simulink model "RoomTemperature"  (R2024a)
settings: Solver=VariableStepAuto  StartTime=0.0  StopTime=T  MaxStep=MaxStep  RelTol=RelTol
values from neighbouring files (symbols this model uses):
  J = 20    [Init.m]
  parameters = [a;Tr;Tdelta;Tmin;Tmax]    [Init.m]
  T = 10    [Init.m]
  xInitial = 55    [Init.m]
  xInitialFsm = 0    [Init.m]
libraries: HyEQ_Library x2, SignalEditorBlockLib x1
settings Model: Creator=venkat  LastModifiedBy=venkat

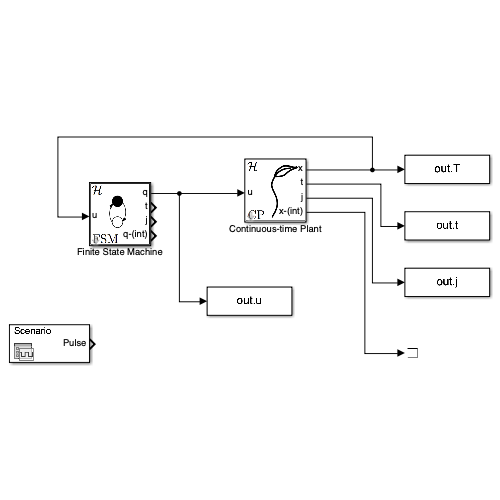
[thumbnail: Simulink's stored preview of the top-level diagram]
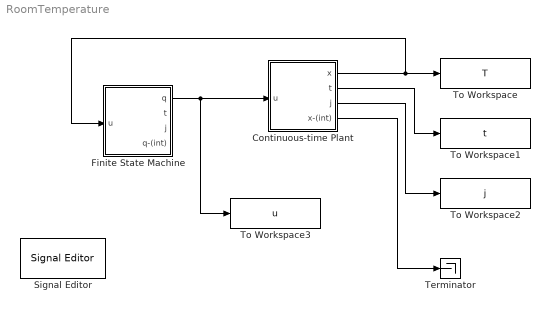
== system RoomTemperature ==
  Continuous-time Plant : Subsystem  LoadFcn=set_param(gcb,'LinkStatus','none')  mask(Continuous Process){z0=xInitial, input_dim=1, parameters=parameters, T=T}
      mask prompts: z0 "Initial State (column vector)"; input_dim "Input dimension (nonnegative integer)"; T "Flow Horizon (nonnegative real)"
      mask help:
      | To define the continuous process:
      | 1. Select the block,
      | 2. "Look inside" the block: Either open the context menu and select Mask > Look Under Mask, or click the arrow in the bottom-left corner of the block.
      | 3. Edit the "flow map f" block to define the continuous dynamics.
      | 4. Edit the "flow set C" block to define the region where the continuous process is allowed to flow.
      mask init:
      | state_dim = size(z0, 1);
      settings: CopyFcn=|
      | set_param(gcb,'LinkStatus','none'),
      | set_param(gcs, 'MaxStep', 'MaxStep', 'RelTol', 'RelTol','StopTime', 'T')
      mask Help: eval hybrid.internal.openHelp('Example_vehicle_on_path')
      mask TypeOptions T: Integrator System/T
      mask DialogControl Control2 Prompt: CPS Components Documentation
      mask DialogControl Control2 Callback: hybrid.internal.openHelp('CPS_Components')
      mask DialogControl ParameterGroupVar Prompt: Configuration
      mask Display:
      | image('Cplant.jpg')
      | port_label('output', 1, 'x')
      | port_label('output', 2, 't')
      | port_label('output', 3, 'j')
      | port_label('output', 4, 'x-(int)')
      | port_label('input', 1, 'u')
  Finite State Machine : Subsystem  LoadFcn=set_param(gcb,'LinkStatus','none')  mask(Finite State Machine (FSM)){q0=xInitialFsm, input_dim=1, T=T, J=J}
      mask prompts: q0 "Initial state (column vector)"; input_dim "Input dimension (nonnegative integer)"; T "Flow Horizon (nonnegative real)"; J "Jump Horizon (nonnegative integer)"
      mask help:
      | To define the FSM:
      | 1. Select the block,
      | 2. "Look inside" the block: Either open the context menu and select Mask > Look Under Mask, or click the arrow in the bottom-left corner of the block.
      | 3. Edit the flow set C, jump set D, and jump map g.
      mask init:
      | state_dim = numel(q0);
      settings: CopyFcn=|
      | set_param(gcb,'LinkStatus','none'),
      | set_param(gcs, 'MaxStep', 'MaxStep', 'RelTol', 'RelTol','StopTime', 'T')
      mask Help: eval hybrid.internal.openHelp('CPS_finite_state_machine')
      mask TypeOptions T: Integrator System/T
      mask TypeOptions J: Integrator System/J
      mask DialogControl Control2 Prompt: CPS Components Documentation
      mask DialogControl Control2 Callback: hybrid.internal.openHelp('CPS_Components')
      mask DialogControl Container4 Prompt: Configuration
      mask Display:
      | image('FSM.jpg')
      | port_label('output', 1, 'q')
      | port_label('output', 2, 't')
      | port_label('output', 3, 'j')
      | port_label('output', 4, 'q-(int)')
      | port_label('input', 1, 'u')
  Signal Editor : SignalEditorBlockLib/Signal Editor  FileName=pulse_signal.mat  ActiveScenario=Scenario  ActiveSignal=Pulse  IsBus=off  OutputBusObjectStr=Bus: BusObject  SampleTime=0  Interpolate=off  ZeroCross=off  OutputAfterFinalValue=Setting to zero  Unit=inherit  PreserveSignalName=on  ApplySigPropsToAllScenarios=on  ApplySigPropsToAllSignals=off
  Terminator : Terminator
  To Workspace : ToWorkspace  VariableName=T  SampleTime=-1
  To Workspace1 : ToWorkspace  VariableName=t  SampleTime=-1
  To Workspace2 : ToWorkspace  VariableName=j  SampleTime=-1
  To Workspace3 : ToWorkspace  VariableName=u  SampleTime=-1
  wires:
  Continuous-time Plant/1(x) -> Finite State Machine/1(u), To Workspace/1
  Continuous-time Plant/2(t) -> To Workspace1/1
  Continuous-time Plant/3(j) -> To Workspace2/1
  Continuous-time Plant/4(x-(int)) -> Terminator/1
  Finite State Machine/1(q) -> To Workspace3/1, Continuous-time Plant/1(u)

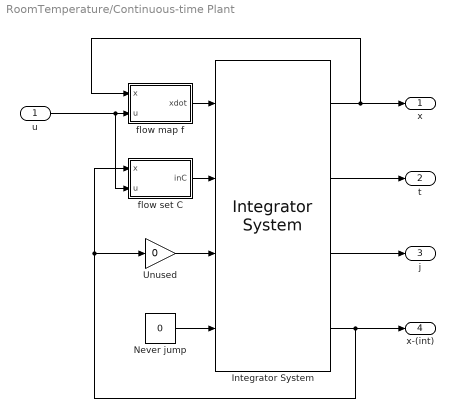
== system RoomTemperature/Continuous-time Plant ==
  u : Inport  PortDimensions=input_dim
  Integrator System : HyEQ_Library/Other/Integrator System  Priority=2  T=T  J=1  x0=z0  rule=1
      settings: SourceProductName=Hybrid Equations Toolbox
  Never jump : Constant  Value=0
  Unused : Gain  Gain=0
  flow map f : MATLAB Function  TreatAsAtomicUnit=on
  flow set C : MATLAB Function  TreatAsAtomicUnit=on
  x : Outport  PortDimensions=state_dim
  t : Outport  Port=2  PortDimensions=1
  j : Outport  Port=3  PortDimensions=1
  x-(int) : Outport  Port=4  PortDimensions=state_dim
  wires:
  Unused/1 -> Integrator System/3
  Never jump/1 -> Integrator System/4
  u/1 -> flow map f/2(u), flow set C/2(u)
  Integrator System/3 -> j/1
  Integrator System/2 -> t/1
  flow set C/1(inC) -> Integrator System/2
  Integrator System/1 -> x/1, flow map f/1(x)
  Integrator System/4 -> x-(int)/1, flow set C/1(x), Unused/1
  flow map f/1(xdot) -> Integrator System/1

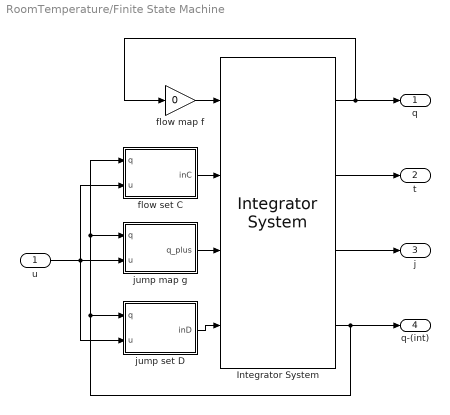
== system RoomTemperature/Finite State Machine ==
  u : Inport  PortDimensions=input_dim
  Integrator System : HyEQ_Library/Other/Integrator System  Priority=2  T=T  J=J  x0=q0  rule=1
      settings: SourceProductName=Hybrid Equations Toolbox
  flow map f : Gain  Gain=0
  flow set C : MATLAB Function  TreatAsAtomicUnit=on
  jump map g : MATLAB Function  TreatAsAtomicUnit=on
  jump set D : MATLAB Function  TreatAsAtomicUnit=on
  q : Outport  PortDimensions=state_dim
  t : Outport  Port=2  PortDimensions=1
  j : Outport  Port=3  PortDimensions=1
  q-(int) : Outport  Port=4  PortDimensions=state_dim
  wires:
  jump map g/1(q_plus) -> Integrator System/3
  jump set D/1(inD) -> Integrator System/4
  u/1 -> jump map g/2(u), jump set D/2(u), flow set C/2(u)
  Integrator System/3 -> j/1
  Integrator System/2 -> t/1
  flow set C/1(inC) -> Integrator System/2
  Integrator System/1 -> q/1, flow map f/1
  Integrator System/4 -> q-(int)/1, flow set C/1(q), jump map g/1(q), jump set D/1(q)
  flow map f/1 -> Integrator System/1

== matlab function RoomTemperature/Finite State Machine/flow set C ==
  data: q input size=state_dim; u input size=input_dim; inC output size=1
function inC  = C(q, u) 
    % Flow set indicator function for finite state machine.
    
    % Specify conditions for when the system should flow.
    inC = 1;
end

== matlab function RoomTemperature/Finite State Machine/jump map g ==
  data: q input size=state_dim; u input size=input_dim; q_plus output size=state_dim
function q_plus = g(q, u)
    % Jump map for finite state machine.
    q_plus = 1-q; 
end

== matlab function RoomTemperature/Finite State Machine/jump set D ==
  data: q input size=state_dim; u input size=input_dim; inD output size=1; parameters parameter
function inD  = D(q, u, parameters) 
    tmin = parameters(4);
    tmax = parameters(5);

    if (q==0 && u<=tmin) || (q==1 && u>=tmax)
        inD = 1
    else
        inD = 0
    end
end

== matlab function RoomTemperature/Continuous-time Plant/flow map f ==
  data: x input size=state_dim; xdot output size=state_dim; u input size=input_dim; parameters parameter
function xdot = f(x, u, parameters)
    % Define the flow map for the continuous process here.
    a = parameters(1);
    Tr = parameters(2);
    Tdelta = parameters(3);

    %eq.
    Tdot = -a*x + Tr + (Tdelta*u);
    xdot = Tdot;
end

== matlab function RoomTemperature/Continuous-time Plant/flow set C ==
  data: x input size=state_dim; inC output size=1; u input size=input_dim
function inC = C(x, u)
    % Define the flow set indicator function for the continuous process here.
    inC = 1;
end
